simulink model "safe_Modif_pto_RM3_copy2"  (R2017b)
settings: Solver=ode4  StartTime=0  StopTime=100000  FixedStep=0.1  MaxStep=0.1  RelTol=1e-3  EnableMultiTasking=on
model workspace (MAT data in the model file):
  p1 = Simulink.Signal
  p1.DataType = 'double'
  p1.Dimensions = -1
  p1.DimensionsMode = 'auto'
  p1.Complexity = 'auto'
  p1.SampleTime = -1
  p1.SamplingMode = 'auto'
values from neighbouring files (symbols this model uses):
  epsilon_int = 0.9    [safe_RealTime_modif22.m]
  m = min(Out,[],2)    [safe_RealTime_modif22.m]
  N_min_eps = 7    [safe_RealTime_modif22.m]
  pnum = 1    [safe_RealTime_modif22.m]
  s = tf('s')    [safe_StateExtraction.m]
  Ts = states_space( state_idx,2)    [safe_RealTime_modif22.m]    (also in safe_StateExtraction.m = TsVec(ts))
undefined symbols (not defined in the file or in its folder): body, constraint, epsilon_thresh, pto, X, Y, Z
libraries: nesl_utility x9, sm_lib x5, WECSim_Lib x4, dspindex x2, dspstat3 x1
settings Model: Creator=mlawson  LastModifiedBy=ghleila
settings SolverCC: ZeroCrossControl=DisableAll  AlgebraicLoopSolver=LineSearch  AutoInsertRateTranBlk=on
settings DataIOCC: SaveFormat=Array  SaveOutput=off  SaveTime=off
settings OptimizationCC: LifeSpan=inf  SimCompilerOptimization=on
settings DebuggingCC: UnderspecifiedInitializationDetection=Classic  MergeDetectMultiDrivingBlocksExec=none  SolverPrmCheckMsg=warning  MultiTaskDSMMsg=none  AllowSymbolicDim=off  StateNameClashWarn=warning  SFUnexpectedBacktrackingDiag=warning  SFNoUnconditionalDefaultTransitionDiag=warning  SFExecutionAtInitializationDiag=none
settings HardwareCC: ProdBitPerPointer=32  ProdBitPerSizeT=32  ProdBitPerPtrDiffT=32  ProdLargestAtomicFloat=None  ProdIntDivRoundTo=Undefined  ProdEndianess=Unspecified  ProdWordSize=32  ProdHWDeviceType=32-bit Generic
settings ModelReferenceCC: PropagateSignalLabelsOutOfModel=off
settings CodeAppCC: StateflowObjectComments=on
settings GRTTargetCC: TargetLangStandard=C89/C90 (ANSI)  GeneratePreprocessorConditionals=Disable all
settings ConfigComp: CovMetricSettings=dw  CovHtmlReporting=on  CovSaveCumulativeToWorkspaceVar=on  CovSaveSingleToWorkspaceVar=on  CovExternalEMLEnable=off  CovSFcnEnable=off
settings SimscapeCC: SimscapeNormalizeSystem=off
settings ExplorerConfigSet: SimMechanicsOpenEditorOnUpdate=off

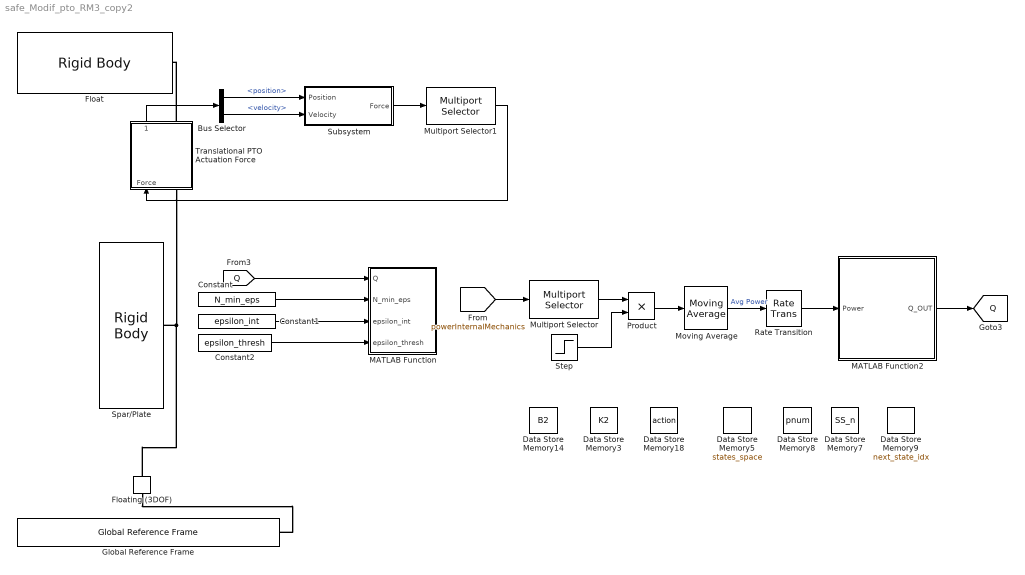
== system safe_Modif_pto_RM3_copy2 ==
  Bus Selector : BusSelector  OutputSignals=position,velocity
  Constant : Constant  Value=N_min_eps
  Constant1 : Constant  Value=epsilon_int
  Constant2 : Constant  Value=epsilon_thresh
  Data Store Memory14 : DataStoreMemory  DataStoreName=B2  ReadBeforeWriteMsg=warning  WriteAfterWriteMsg=warning  WriteAfterReadMsg=warning  InitialValue=2000000  ShareAcrossModelInstances=on  VectorParams1D=off  ShowAdditionalParam=off  OutDataTypeStr=double
  Data Store Memory18 : DataStoreMemory  DataStoreName=action  ReadBeforeWriteMsg=warning  WriteAfterWriteMsg=warning  WriteAfterReadMsg=warning  InitialValue=action  VectorParams1D=off  ShowAdditionalParam=off  OutDataTypeStr=double
  Data Store Memory3 : DataStoreMemory  DataStoreName=K2  ReadBeforeWriteMsg=warning  WriteAfterWriteMsg=warning  WriteAfterReadMsg=warning  InitialValue=1000000  ShareAcrossModelInstances=on  ShowAdditionalParam=off  OutDataTypeStr=double
  Data Store Memory5 : DataStoreMemory  DataStoreName=states_space  ReadBeforeWriteMsg=warning  WriteAfterWriteMsg=warning  WriteAfterReadMsg=warning  InitialValue=states_space  VectorParams1D=off  ShowAdditionalParam=off  OutDataTypeStr=double
  Data Store Memory7 : DataStoreMemory  DataStoreName=SS_n  ReadBeforeWriteMsg=warning  WriteAfterWriteMsg=warning  WriteAfterReadMsg=warning  InitialValue=SS_n  VectorParams1D=off  ShowAdditionalParam=off  OutDataTypeStr=double
  Data Store Memory8 : DataStoreMemory  DataStoreName=pnum  ReadBeforeWriteMsg=warning  WriteAfterWriteMsg=warning  WriteAfterReadMsg=warning  ShowAdditionalParam=off  OutDataTypeStr=double
  Data Store Memory9 : DataStoreMemory  DataStoreName=next_state_idx  ReadBeforeWriteMsg=warning  WriteAfterWriteMsg=warning  WriteAfterReadMsg=warning  InitialValue=1  ShowAdditionalParam=off  OutDataTypeStr=double
  Float : WECSim_Lib/Body Elements/Rigid Body  body=body(1)
      settings: AttributesFormatString=%<body>
  Floating (3DOF) : WECSim_Lib/Constraints/Floating (3DOF)  constraint=constraint(1)
      settings: AttributesFormatString=%<constraint>
  Global Reference Frame : WECSim_Lib/Frames/Global Reference Frame  waves=waves  simu=simu
  MATLAB Function : MATLAB Function  TreatAsAtomicUnit=on
  MATLAB Function2 : MATLAB Function  TreatAsAtomicUnit=on
  Moving Average : dspstat3/Moving Average  Method=Sliding window  SpecifyWindowLength=on  WindowLength=20*Ts/0.1  ForgettingFactor=0.9  SimulateUsing=Code generation
  Multiport Selector : dspindex/Multiport Selector  rowsOrCols=Rows  idxCellArray={ 3}  idxErrMode=Clip Index
  Multiport Selector1 : dspindex/Multiport Selector  rowsOrCols=Rows  idxCellArray={ 3}  idxErrMode=Clip Index
  Product : Product
  Rate Transition : RateTransition  OutPortSampleTime=20*Ts
  Spar/Plate : WECSim_Lib/Body Elements/Rigid Body  body=body(2)
      settings: AttributesFormatString=%<body>
  Step : Step  SampleTime=20*(pnum)*Ts
  Subsystem : Subsystem
  Translational PTO Actuation Force : Subsystem  AncestorBlock=WECSim_Lib/PTOs/Translational PTO Actuation Force  mask(PTO){pto=pto(1)}
      mask prompts: pto "PTO Name:"
      mask help:
      | Constraints the follower to translational motion relative to the base, in
      | the PTO's Z-direction and adds PTO stiffness and damping. Also applies a
      | user-defined force and outputs extension, velocity, and acceleration.
      |
      |
      | The variable name input below must be 'pto(i)' where i=1,2,...
      | pto(i) must be defined in the input file with the following fields:
      |
      |     .name (required)
      |             String.
      |             PTO name. Must comply with Matlab's variable naming rules.
      |     .loc (optional)
      |             3x1 vector [x y z] in meters.
      |             PTO location. Default = [0 0 0]
      |     .k (optional)
      |             Float.
      |             PTO linear spring stiffness. Default = 0
      |     .c (optional)
      |             Float.
      |             PTO linear damping coefficient. Default = 0
      |     .orientation.z (optional)
      |             3x1 vector [x y z].
      |             Direction of the PTO's Z-coordinate. Default = [0 0 1]
      |     .orientation.y (optional)
      |             3x1 vector [x y z].
      |             Direction of the PTO's Y-coordinate. Default = [0 1 0]
      mask init:
      | if exist('pto','var')
      |     h=[gcb '/output'];
      |     responseName=['pto' num2str(pto.ptoNum) '_out'];
      |     set_param(h,'VariableName',responseName);
      | end
      | 
      | pto.checkLoc('W');
      settings: AttributesFormatString=%<pto>
      mask Help:
      | Constraints the follower to translational motion relative to the base, in
      | the PTO's Z-direction and adds PTO stiffness and damping. Also applies a
      | user-defined force and outputs extension, velocity, and acceleration.
      | 
      | 
      | The variable name input below must be 'pto(i)' where i=1,2,...
      | pto(i) must be defined in the input file with the following fields:
      | 
      |     .name (required)
      |             String.
      |             PTO name. Must comply with Matlab's variable naming rules.
      |     .loc (optional)
      |             3x1 vector [x y z] in meters.
      |             PTO location. Default = [0 0 0]
      |     .k (optional)
      |             Float.
      |             PTO linear spring stiffness. Default = 0
      |     .c (optional)
      |             Float.
      |             PTO linear damping coefficient. Default = 0
      |     .orientation.z (optional)
      |             3x1 vector [x y z].
      |             Direction of the PTO's Z-coordinate. Default = [0 0 1]
      |     .orientation.y (optional)
      |             3x1 vector [x y z].
      |             Direction of the PTO's Y-coordinate. Default = [0 1 0]
  tag scope: Q=global
  wires:
  Multiport Selector/1 -> Product/1
  [powerInternalMechanics] -> Multiport Selector/1
  Moving Average/1 -> Rate Transition/1  "Avg Power"
  Translational PTO Actuation Force/1(Response) -> Bus Selector/1
  Bus Selector/2 -> Subsystem/2(Velocity)  "<velocity>"
  Bus Selector/1 -> Subsystem/1(Position)  "<position>"
  Subsystem/1(Force) -> Multiport Selector1/1
  Multiport Selector1/1 -> Translational PTO Actuation Force/1(Force)
  Product/1 -> Moving Average/1
  Step/1 -> Product/2
  [Q] -> MATLAB Function/1(Q)
  MATLAB Function2/1(Q_OUT) -> [Q]
  Rate Transition/1 -> MATLAB Function2/1(Power)
  Constant/1 -> MATLAB Function/2(N_min_eps)
  Constant1/1 -> MATLAB Function/3(epsilon_int)
  Constant2/1 -> MATLAB Function/4(epsilon_thresh)
  connections:
  Floating (3DOF)/RConn1 -- Translational PTO Actuation Force/LConn1 -- Spar/Plate/RConn1
  Floating (3DOF)/LConn1 -- Global Reference Frame/RConn1
  Translational PTO Actuation Force/RConn1 -- Float/RConn1

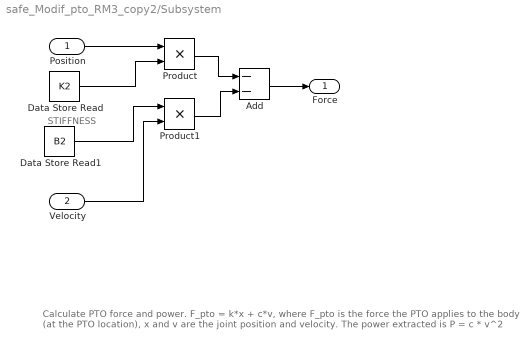
== system safe_Modif_pto_RM3_copy2/Subsystem ==
  note: STIFFNESS
  note: Calculate PTO force and power.
      |
      | F_pto  = k*x + c*v,
      | where F_pto is the force the PTO applies to the body (at the PTO location), x and v are the joint position and velocity.
      |
      | The power extracted is
      | P = c * v^2
  Position : Inport
  Velocity : Inport  Port=2
  Add : Sum  Inputs=--
  Data Store Read : DataStoreRead  DataStoreName=K2
  Data Store Read1 : DataStoreRead  DataStoreName=B2
  Product : Product  Inputs=**
  Product1 : Product  Inputs=**
  Force : Outport
  wires:
  Add/1 -> Force/1
  Product/1 -> Add/1
  Data Store Read1/1 -> Product1/1
  Velocity/1 -> Product1/2
  Product1/1 -> Add/2
  Data Store Read/1 -> Product/2
  Position/1 -> Product/1

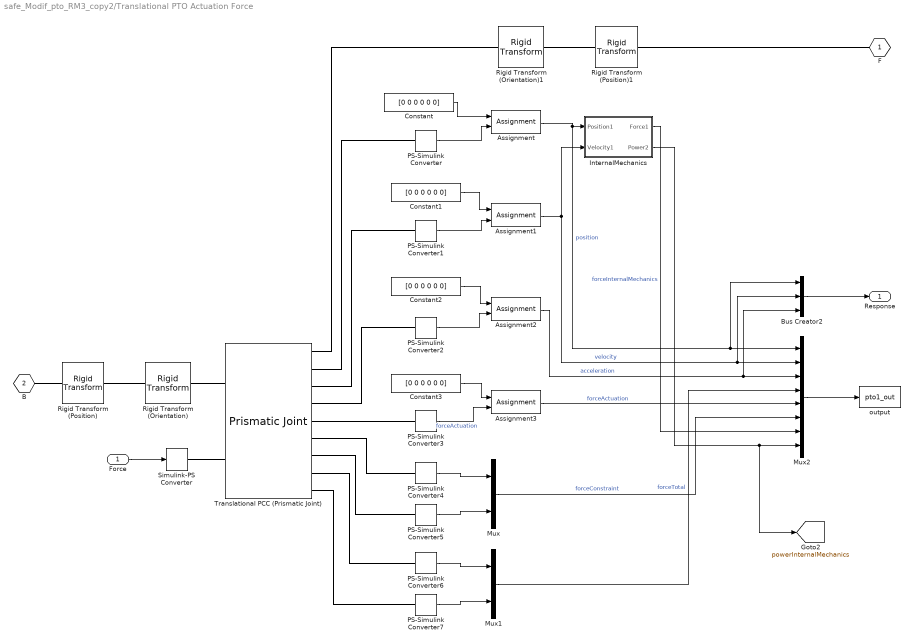
== system safe_Modif_pto_RM3_copy2/Translational PTO Actuation Force ==
  Force : Inport
  Assignment{,1..3} (4 alike) : Assignment  IndexOptions=Index vector (dialog)  Indices=3  OutputSizes=1
  Bus Creator2 : BusCreator  Inputs=3
  Constant{,1..3} (4 alike) : Constant  Value=[0 0 0 0 0 0]
  InternalMechanics : Subsystem
  Mux : Mux  Inputs=2
  Mux1 : Mux  Inputs=2
  Mux2 : Mux  Inputs=8
  PS-Simulink Converter{,1..7} (8 alike) : nesl_utility/PS-Simulink Converter  PhysicalDomain=network_engine_domain  SubClassName=ps_output  LeftPortType=input  RightPortType=output  PseudoPeriodic=off  Frequencies=[]  Unit=1  AffineConversion=off
  Rigid Transform (Position) : sm_lib/Frames and Transforms/Rigid Transform  TranslationMethod=Cartesian  TranslationStandardOffset=0  TranslationLengthUnit=m  TranslationStandardAxis=+Z  TranslationCartesianOffset=pto.initDisp.initLinDisp + pto.loc  TranslationROffset=0  TranslationROffsetUnits=m  TranslationZOffset=0  TranslationZOffsetUnits=m  TranslationThetaOffset=0  TranslationThetaOffsetUnits=deg  RotationMethod=None  RotationAngleUnits=rad  RotationStandardAxis=+Y  RotationAngle=0  RotationArbitraryAxis=[0 1 0]  FollAlignAxisA=+X  BaseAlignAxisA=+Y  FollAlignAxisB=+Y  BaseAlignAxisB=+Z  RotationSequenceAxes=FollowerAxes  RotationSequence=XYX  RotationSequenceAngles=[0 0 0]  RotationSequenceAnglesUnits=deg  RotationMatrix=[1 0 0; 0 1 0; 0 0 1]
  Rigid Transform (Position)1 : sm_lib/Frames and Transforms/Rigid Transform  TranslationMethod=Cartesian  TranslationStandardOffset=0  TranslationLengthUnit=m  TranslationStandardAxis=+Z  TranslationCartesianOffset=pto.initDisp.initLinDisp + pto.loc  TranslationROffset=0  TranslationROffsetUnits=m  TranslationZOffset=0  TranslationZOffsetUnits=m  TranslationThetaOffset=0  TranslationThetaOffsetUnits=deg  RotationMethod=None  RotationAngleUnits=rad  RotationStandardAxis=+Y  RotationAngle=0  RotationArbitraryAxis=[0 1 0]  FollAlignAxisA=+X  BaseAlignAxisA=+Y  FollAlignAxisB=+Y  BaseAlignAxisB=+Z  RotationSequenceAxes=FollowerAxes  RotationSequence=XYX  RotationSequenceAngles=[0 0 0]  RotationSequenceAnglesUnits=deg  RotationMatrix=[1 0 0; 0 1 0; 0 0 1]
  Rigid Transform (Orientation) : sm_lib/Frames and Transforms/Rigid Transform  TranslationMethod=None  TranslationStandardOffset=0  TranslationLengthUnit=m  TranslationStandardAxis=+Z  TranslationCartesianOffset=0  TranslationROffset=0  TranslationROffsetUnits=m  TranslationZOffset=0  TranslationZOffsetUnits=m  TranslationThetaOffset=0  TranslationThetaOffsetUnits=deg  RotationMethod=RotationMatrix  RotationAngleUnits=rad  RotationStandardAxis=+Y  RotationAngle=0  RotationArbitraryAxis=[0 1 0]  FollAlignAxisA=+X  BaseAlignAxisA=+Y  FollAlignAxisB=+Y  BaseAlignAxisB=+Z  RotationSequenceAxes=FollowerAxes  RotationSequence=XYX  RotationSequenceAngles=[0 0 0]  RotationSequenceAnglesUnits=deg  RotationMatrix=pto.orientation.rotationMatrix
  Rigid Transform (Orientation)1 : sm_lib/Frames and Transforms/Rigid Transform  TranslationMethod=None  TranslationStandardOffset=0  TranslationLengthUnit=m  TranslationStandardAxis=+Z  TranslationCartesianOffset=0  TranslationROffset=0  TranslationROffsetUnits=m  TranslationZOffset=0  TranslationZOffsetUnits=m  TranslationThetaOffset=0  TranslationThetaOffsetUnits=deg  RotationMethod=RotationMatrix  RotationAngleUnits=rad  RotationStandardAxis=+Y  RotationAngle=0  RotationArbitraryAxis=[0 1 0]  FollAlignAxisA=+X  BaseAlignAxisA=+Y  FollAlignAxisB=+Y  BaseAlignAxisB=+Z  RotationSequenceAxes=FollowerAxes  RotationSequence=XYX  RotationSequenceAngles=[0 0 0]  RotationSequenceAnglesUnits=deg  RotationMatrix=pto.orientation.rotationMatrix
  Simulink-PS Converter : nesl_utility/Simulink-PS Converter  PhysicalDomain=network_engine_domain  SubClassName=ps_input  LeftPortType=input  RightPortType=output  PseudoPeriodic=off  Frequencies=[]  NoiseDistribution=none  NoiseParameters=[]  Unit=1  AffineConversion=off  FilteringAndDerivatives=zero  SimscapeFilterOrder=1  InputFilterTimeConstant=0.001  UdotUserProvided=1
  Translational PCC (Prismatic Joint) : sm_lib/Joints/Prismatic Joint  SenseConstraintForce=on  SenseConstraintForceX=off  SenseConstraintForceY=off  SenseConstraintForceZ=off  SenseConstraintTorque=on  SenseConstraintTorqueX=off  SenseConstraintTorqueY=off  SenseConstraintTorqueZ=off  SenseTotalForce=on  SenseTotalForceX=off  SenseTotalForceY=off  SenseTotalForceZ=off  SenseTotalTorque=on  SenseTotalTorqueX=off  SenseTotalTorqueY=off  SenseTotalTorqueZ=off  CompositeWrenchDir=BaseOnFollower  CompositeWrenchFrame=BaseFrame  EquilibriumPosition=0  EquilibriumPositionUnits=m  SpringStiffness=pto.k  SpringStiffnessUnits=N/m  DampingCoefficient=pto.c  DampingCoefficientUnits=N/(m/s)  TorqueActuationMode=InputTorque  MotionActuationMode=ComputedMotion  SensePosition=on  SenseVelocity=on  SenseAcceleration=on  SenseTorqueForce=on  PositionTargetSpecify=off  PositionTargetPriority=High  PositionTargetValue=0  PositionTargetValueUnits=m  VelocityTargetSpecify=off  VelocityTargetPriority=High  VelocityTargetValue=0  VelocityTargetValueUnits=m/s
  output : ToWorkspace  VariableName=pto1_out  SaveFormat=Structure With Time  SampleTime=-1
      settings: Decimation=round(simu.dtOut/simu.dt,0)
  F : PMIOPort  Port=1  Side=Right
  B : PMIOPort  Port=2  Side=Left
  Response : Outport
  tag scope: powerInternalMechanics=global
  wires:
  Bus Creator2/1 -> Response/1
  Assignment/1 -> InternalMechanics/1(Position1), Mux2/1, Bus Creator2/1  "position"
  Assignment1/1 -> InternalMechanics/2(Velocity1), Mux2/2, Bus Creator2/2  "velocity"
  Assignment2/1 -> Mux2/3, Bus Creator2/3  "acceleration"
  Force/1 -> Simulink-PS Converter/1
  Mux2/1 -> output/1
  Mux/1 -> Mux2/6  "forceConstraint"
  Mux1/1 -> Mux2/4  "forceTotal"
  PS-Simulink Converter4/1 -> Mux/1
  PS-Simulink Converter5/1 -> Mux/2
  PS-Simulink Converter6/1 -> Mux1/1
  PS-Simulink Converter7/1 -> Mux1/2
  Assignment3/1 -> Mux2/5  "forceActuation"
  Constant/1 -> Assignment/1
  PS-Simulink Converter/1 -> Assignment/2
  Constant1/1 -> Assignment1/1
  PS-Simulink Converter1/1 -> Assignment1/2
  Constant2/1 -> Assignment2/1
  PS-Simulink Converter2/1 -> Assignment2/2
  Constant3/1 -> Assignment3/1
  PS-Simulink Converter3/1 -> Assignment3/2  "forceActuation"
  InternalMechanics/1(Force1) -> Mux2/7  "forceInternalMechanics"
  InternalMechanics/2(Power2) -> [powerInternalMechanics], Mux2/8
  connections:
  Rigid Transform (Position)/RConn1 -- Rigid Transform (Orientation)/LConn1
  Rigid Transform (Position)1/RConn1 -- Rigid Transform (Orientation)1/LConn1
  Simulink-PS Converter/RConn1 -- Translational PCC (Prismatic Joint)/LConn2
  Rigid Transform (Orientation)/RConn1 -- Translational PCC (Prismatic Joint)/LConn1
  Rigid Transform (Position)/LConn1 -- B/RConn1
  Translational PCC (Prismatic Joint)/RConn5 -- PS-Simulink Converter3/LConn1
  Translational PCC (Prismatic Joint)/RConn9 -- PS-Simulink Converter7/LConn1
  Rigid Transform (Orientation)1/RConn1 -- Translational PCC (Prismatic Joint)/RConn1
  Translational PCC (Prismatic Joint)/RConn4 -- PS-Simulink Converter2/LConn1
  Translational PCC (Prismatic Joint)/RConn7 -- PS-Simulink Converter5/LConn1
  Translational PCC (Prismatic Joint)/RConn3 -- PS-Simulink Converter1/LConn1
  Rigid Transform (Position)1/LConn1 -- F/RConn1
  Translational PCC (Prismatic Joint)/RConn8 -- PS-Simulink Converter6/LConn1
  Translational PCC (Prismatic Joint)/RConn2 -- PS-Simulink Converter/LConn1
  Translational PCC (Prismatic Joint)/RConn6 -- PS-Simulink Converter4/LConn1

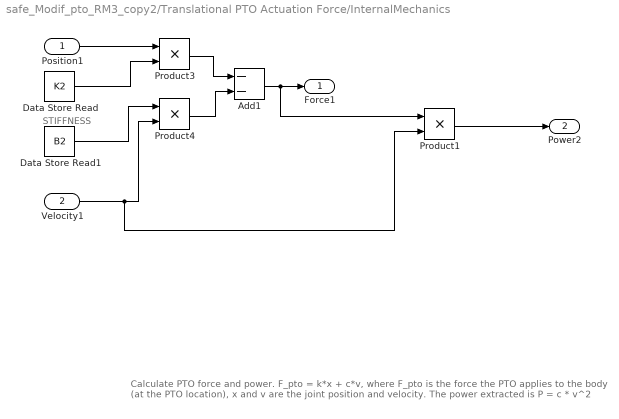
== system safe_Modif_pto_RM3_copy2/Translational PTO Actuation Force/InternalMechanics ==
  note: Calculate PTO force and power.
      |
      | F_pto  = k*x + c*v,
      | where F_pto is the force the PTO applies to the body (at the PTO location), x and v are the joint position and velocity.
      |
      | The power extracted is
      |
      | P = c * v^2
  note: STIFFNESS
  Position1 : Inport
  Velocity1 : Inport  Port=2
  Add1 : Sum  Inputs=--
  Data Store Read : DataStoreRead  DataStoreName=K2
  Data Store Read1 : DataStoreRead  DataStoreName=B2
  Product1 : Product  Inputs=**
  Product3 : Product  Inputs=**
  Product4 : Product  Inputs=**
  Force1 : Outport
  Power2 : Outport  Port=2
  wires:
  Product3/1 -> Add1/1
  Product4/1 -> Add1/2
  Velocity1/1 -> Product1/2, Product4/2
  Data Store Read/1 -> Product3/2
  Add1/1 -> Product1/1, Force1/1
  Data Store Read1/1 -> Product4/1
  Position1/1 -> Product3/1
  Product1/1 -> Power2/1

== matlab function safe_Modif_pto_RM3_copy2/MATLAB Function ==
  data: action data_store_memory; states_space data_store_memory; Q input; B2 data_store_memory; K2 data_store_memory; next_state_idx data_store_memory; N_min_eps input; epsilon_int input; epsilon_thresh input
function fcn1(Q,N_min_eps,epsilon_int,epsilon_thresh)

global action states_space B2 K2 next_state_idx
persistent ove_count state_idx N_epsilon

%% initial state


if isempty (ove_count)
    ove_count=1;
else
    ove_count=ove_count+1;
end

if isempty (state_idx)
    state_idx=1;
end

if isempty (Q)
    Q=rand(size(states_space,1),size(states_space,2));
end


if isempty (N_epsilon)
    N_epsilon=zeros(size(states_space,1),1);
end


coder.extrinsic('num2str','datasample','get_param','feedforwardnet','train');
disp(['iteration: ' num2str(ove_count)]);


        N_ep=N_epsilon(state_idx,1)-N_min_eps;
        if N_ep>0
            epsilon=epsilon_int/sqrt(N_ep);
            if epsilon<=epsilon_thresh
                epsilon=0;
            end
        else
            epsilon=epsilon_int;
        end
        
        %%% N_epsilon
        N_epsilon(state_idx,1)=N_epsilon(state_idx,1)+1;
        
epsilon
%% taking an action

r=rand; % get 1 uniform random number

x=sum(r>=cumsum([0, 1-epsilon, epsilon])); % check it to be in which probability area
% choose either explore or exploit

if x == 1   % exploit
    
    [~,umax]=max(Q(state_idx,:));
    
    % [~,umax]=max(V(state_idx,1));
    
    current_action = action(umax,:);
    
else        % explore
    
    
    % action_idx=zeros(1,1);
    
    current_action=datasample(action,1); % choose 1 action randomly (uniform random distribution)
end

B2=current_action(1,1);
%
K2=current_action(1,2);

action_idx = find(action(:,1)==B2 & action(:,2)==K2); % id of the chosen action

action_idx=action_idx(1,1);



%% next state
st_chosen=double(0);
st_chosen=datasample(1:size(states_space,1),1); % choose 1 action randomly (uniform random distribution)

Height =states_space( st_chosen,1);           %m         %Amplitude of the waves

Ts =states_space( st_chosen,2);             %s         %Significant period of the Wave


next_state_idx1=find(states_space(:,1)==Height & states_space(:,2)==Ts & states_space(:,3)==B2 & states_space(:,4)==K2);
next_state_idx=next_state_idx1(1,1);

state_idx=next_state_idx;

== matlab function safe_Modif_pto_RM3_copy2/MATLAB Function2 ==
  data: action data_store_memory; states_space data_store_memory; SS_n data_store_memory; Q_OUT output; Power input; next_state_idx data_store_memory; B2 data_store_memory; K2 data_store_memory; pnum data_store_memory
function Q_OUT =fcn1(Power)

global  action  states_space SS_n B2 K2 next_state_idx pnum

persistent Q Q_prime Q_targ Memory_Stor ove_count  MeanR R Final_Rew_matt state_idx num_R N_alpha


Memory_D_size=500;
num_state=size(states_space,1);
num_act=size(action,1);


if isempty (state_idx)
    state_idx=1;

end

if isempty (Q)
    Q=rand(num_state,num_act);
end


if isempty (Q_prime)
    Q_prime=rand(num_state,num_act);
end



if isempty (Q_targ)
    Q_targ=rand(num_state,num_act);
end

if isempty (Final_Rew_matt)
    Final_Rew_matt=zeros(num_state,1);
end
% 
if isempty (Memory_Stor)
    
    Memory_Stor=zeros(5*Memory_D_size,4+size(states_space,2)+size(Q,2));
end



if isempty (ove_count)
    ove_count=1;
else
    ove_count=ove_count+1;
end


if isempty (R)
    R=zeros(num_state,75);
end

if isempty (MeanR)
    MeanR=zeros(num_state,1);
end

if isempty (num_R)
    num_R=zeros(num_state,1);
end

if isempty (N_alpha)
    N_alpha=zeros(size(states_space,1),num_act);
end


PptoAvg=Power;

%% initial values

gamma_int=0.9;   %%% discount factor
alph_int=0.4;  %% learning rate
N_min_alpha=7;
pnum=pnum+1;
gamma=0.7;

PptoAvg=-(Power(1,1)); %% generated power is negative


%% initial state


coder.extrinsic('num2str','datasample','get_param','feedforwardnet','train');


% if ove_count>=150
%     
%     gamma=0.9;
% else
%     
%     gamma=0.6;
%     
% end



%% next_state

action_idx = find(action(:,1)==B2 & action(:,2)==K2);

Height =states_space( next_state_idx,1);           %m         %Amplitude of the waves

Ts =states_space( next_state_idx,2);

        if N_alpha(state_idx,action_idx)-N_min_alpha>0
            alpha=alph_int/N_alpha(state_idx,action_idx);
        else
            alpha=alph_int;
        end

N_alpha(state_idx,action_idx)=N_alpha(state_idx,action_idx)+1;
%% allocating power
num_R(next_state_idx)=num_R(next_state_idx)+1;
next_reward=(PptoAvg/(Height^2)); %% normalized reward

R(next_state_idx,num_R(next_state_idx))=next_reward;
Height=states_space(next_state_idx,1);
Height=Height(1,1);

Period=states_space(next_state_idx,2);
Period=Period(1,1);



R_idx=find(states_space(:,1)==Height& states_space(:,2)==Period);

%%% MeanR from 3rd column of R were chosen to remove the first random and
%%% sometimes inaccurate results

MeanR(R_idx,1)=sum(R(R_idx,3:end),2)./num_R(R_idx) % mean


MaxR=max(MeanR(R_idx));

Final_Rew_matt(R_idx)=MeanR(R_idx,1)/MaxR;

Final_Rew=Final_Rew_matt(next_state_idx);

Final_Rew=(Final_Rew)^5;


%% storing features

% All_features(ove_count,:)=All_params3;  %%% to get an idea about the max of each parameter

disp(['current state : ' num2str(state_idx) ' next state : ' num2str(next_state_idx) ' taken action : ' num2str(action(action_idx,:))]);

disp([' next reward : ' num2str(Final_Rew)]);

%% neural network part


if ove_count> 5  %% start traing network
    
    %% droping off very old data
    
    if ove_count>Memory_D_size %% dropoff
        
        In=Memory_Stor(ove_count-Memory_D_size:ove_count-1,5:8);
        
        Output=Memory_Stor(ove_count-Memory_D_size:ove_count-1,9:end);
        
        nodes = [size(In,2) size(action,1)];
        
    else
        
        In=Memory_Stor(1:ove_count-1,5:8);
        
        Output=Memory_Stor(1:ove_count-1,9:end);
        
        nodes = [size(In,2) size(action,1)];
        
    end

    
    Out=[];
    Out=Output;
    m = min(Out,[],2);
    range = max(Out,[],2) - m;
    Out1=bsxfun(@minus,Out,m);
    Out=bsxfun(@rdivide,Out1,range) ;
    
    Input=[];
    Input=In;
    m11 = min(Input);
    range1 = max(Input) - m11;
    Input=bsxfun(@minus,Input,m11);
    Input=bsxfun(@rdivide,Input,range1) ;
    
    
    %% correction for one sea state
    Input(:,1:2) =ones(size(Input,1),2);
    
    net = feedforwardnet([5]);
    [net,tr] = train(net,Input',Out');
    %
    %
    y_prime= net(SS_n(next_state_idx,:)');
    Q_prime(next_state_idx,:) =y_prime';
    
    Q_targ(state_idx,action_idx)=Final_Rew+gamma*max(Q_prime(next_state_idx,:)); % update q values
    
    target=Q;
    Q_prev=Q;
    
    target(state_idx,action_idx)=Q_targ(state_idx,action_idx); %%% update target
    Memory_Stor(ove_count,:)=[state_idx,action_idx,Final_Rew,next_state_idx,states_space(state_idx,:),target(state_idx,:)];
    result=[state_idx,action_idx,Final_Rew,next_state_idx];
    %% training NN with recent data
    %        [dnn,out_est,rmse]=DNNf(Input,Output,nodes,opts);
    
else
    % Q_prev=Q;
    

     Q(state_idx,action_idx)=Q(state_idx,action_idx)+alpha*(Final_Rew+gamma*max(Q(next_state_idx,:))-Q(state_idx,action_idx));
    target=Q;
    
    Memory_Stor(ove_count,:)=[state_idx,action_idx,Final_Rew,next_state_idx,states_space(state_idx,:),target(state_idx,:)];
end

%% checking the convergence of  Q function

Q=target;

% dif(ove_count)=norm(target(:,:)-Q_prev(:,:),Inf);

ove_count=ove_count+1;
next_state_idx=next_state_idx(1,1);

state_idx=next_state_idx;

Q
Q_OUT=Q;
